simulink model "pidccontrol"  (R2014b)
settings: Solver=VariableStepAuto  StartTime=0.0  StopTime=Tstop  FixedStep=Ts  RelTol=1e-3
values from neighbouring files (symbols this model uses):
  inputnoisegain = 0    [DMCejemplo.m]
  outputnoisegain = 0    [DMCejemplo.m]
  steptimeDV = 35    [DMCejemplo.m]
  steptimeUDV = 45    [DMCejemplo.m]
  Ts = 0.5    [DMCejemplo.m]
  valueDV = 2    [DMCejemplo.m]
  valueUDV = -2    [DMCejemplo.m]
undefined symbols (not defined in the file or in its folder): Kc, Kpre, Ti
undefined symbols (not defined in the file): gdv, gu, gudv
libraries: cstblocks x3, simulink x2
settings Model: Creator=juaherdu  LastModifiedBy=juaherdu
settings DataIOCC: SaveFormat=Dataset
settings OptimizationCC: UseDivisionForNetSlopeComputation=off  SimCompilerOptimization=off
settings DebuggingCC: SolverPrmCheckMsg=none  FrameProcessingCompatibilityMsg=error  AllowSymbolicDim=off
settings HardwareCC: ProdBitPerPointer=64  ProdLargestAtomicFloat=Float  ProdIntDivRoundTo=Zero  ProdEndianess=LittleEndian  ProdWordSize=64  ProdHWDeviceType=Intel->x86-64 (Windows64)
settings RTWCC: RTWCompilerOptimization=off
settings GRTTargetCC: GeneratePreprocessorConditionals=Use local settings
settings ConfigComp: CovMetricSettings=dw  CovHtmlReporting=on  CovSaveCumulativeToWorkspaceVar=on  CovSaveSingleToWorkspaceVar=on  CovExternalEMLEnable=off

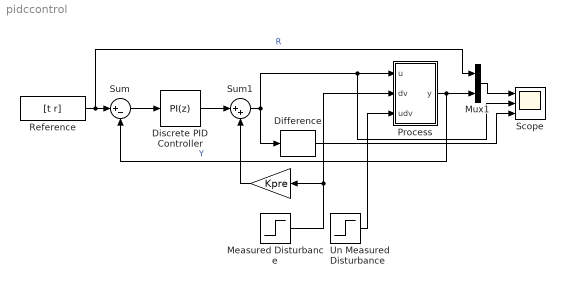
== system pidccontrol ==
  " " : Gain  Gain=Kpre
  Difference : simulink/Discrete/Difference  ICPrevInput=0.0  InputProcessing=Inherited  OutMin=[]  OutMax=[]  OutDataType=fixdt(1, 16)  OutScaling=2^-10  DoSatur=off
  Discrete PID Controller : simulink/Continuous/PID Controller  Controller=PI  TimeDomain=Discrete-time  SampleTime=Ts  IntegratorMethod=Forward Euler  FilterMethod=Forward Euler  Form=Ideal  P=Kc  I=1/Ti  D=0  N=100  InitialConditionSource=internal  InitialConditionForIntegrator=0  InitialConditionForFilter=0  ExternalReset=none  LimitOutput=off  UpperSaturationLimit=inf  LowerSaturationLimit=-inf  LinearizeAsGain=on  AntiWindupMode=none  Kb=1  TrackingMode=off  Kt=1  PParamMin=[]  PParamMax=[]  IParamMin=[]  IParamMax=[]  DParamMin=[]  DParamMax=[]  NParamMin=[]  NParamMax=[]  KbParamMin=[]  KbParamMax=[]  KtParamMin=[]  KtParamMax=[]  POutMin=[]  POutMax=[]  IOutMin=[]  IOutMax=[]  DOutMin=[]  DOutMax=[]  NOutMin=[]  NOutMax=[]  KbOutMin=[]  KbOutMax=[]  KtOutMin=[]  KtOutMax=[]  IntegratorOutMin=[]  IntegratorOutMax=[]  FilterOutMin=[]  FilterOutMax=[]  SumOutMin=[]  SumOutMax=[]  SumI1OutMin=[]  SumI1OutMax=[]  SumI2OutMin=[]  SumI2OutMax=[]  SumI3OutMin=[]  SumI3OutMax=[]  SumDOutMin=[]  SumDOutMax=[]  SaturationOutMin=[]  SaturationOutMax=[]  IntegratorContinuousStateAttributes=''  IntegratorStateMustResolveToSignalObject=off  IntegratorRTWStateStorageClass=Auto  FilterContinuousStateAttributes=''  FilterStateMustResolveToSignalObject=off  FilterRTWStateStorageClass=Auto  DifferentiatorICPrevScaledInput=0  DifferentiatorOutMin=[]  DifferentiatorOutMax=[]  UseFilter=on
  Measured Disturbance : Step  Time=steptimeDV  After=valueDV  SampleTime=Ts
  Mux1 : Mux  Inputs=2
  Process : Subsystem  mask{gu=gu, gdv=gdv, gudv=gudv, inputnoisegain=inputnoisegain, outputnoisegain=outputnoisegain}
      mask prompts: gu "fdt y/u"; gdv "fdt y/dv"; gudv "fdt y/udv"; inputnoisegain "inputnoise"; outputnoisegain "outputnoise"
      mask DialogControl DescTextVar Prompt: Parametros del Modelo del proceso
  Reference : FromWorkspace  VariableName=[t r]  SampleTime=Ts
  Scope : Scope  NumInputPorts=3
      settings: ShowLegends=on  YMin=-1.61853~-1.61915~-0.12834  YMax=14.56673~14.57238~0.68093  SaveName=Simul  MaxDataPoints=50000
  Sum : Sum  Inputs=|+-
  Sum1 : Sum  Inputs=|++
  Un Measured Disturbance : Step  Time=steptimeUDV  After=valueUDV  SampleTime=Ts
  wires:
  Measured Disturbance/1 -> " "/1, Process/2(dv)
  Un Measured Disturbance/1 -> Process/3(udv)
  Reference/1 -> Mux1/1, Sum/1  "R"
  Sum1/1 -> Scope/2, Process/1(u), Difference/1
  Process/1(y) -> Sum/2, Mux1/2  "Y"
  Mux1/1 -> Scope/1
  Difference/1 -> Scope/3
  Sum/1 -> Discrete PID Controller/1
  Discrete PID Controller/1 -> Sum1/1
  " "/1 -> Sum1/2

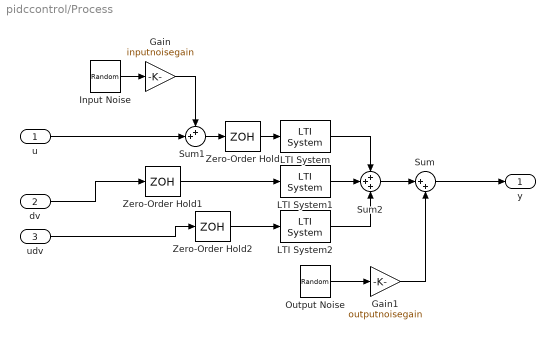
== system pidccontrol/Process ==
  u : Inport
  dv : Inport  Port=2
  udv : Inport  Port=3
  Gain : Gain  Gain=inputnoisegain
  Gain1 : Gain  Gain=outputnoisegain
  Input Noise : UniformRandomNumber  SampleTime=Ts
  LTI System : cstblocks/LTI System  sys=gu  IC=[]
  LTI System1 : cstblocks/LTI System  sys=gdv  IC=[]
  LTI System2 : cstblocks/LTI System  sys=gudv  IC=[]
  Output Noise : UniformRandomNumber  SampleTime=Ts
  Sum : Sum  Inputs=|++
  Sum1 : Sum  Inputs=++|
  Sum2 : Sum  Inputs=+++
  Zero-Order Hold : ZeroOrderHold  SampleTime=Ts
  Zero-Order Hold1 : ZeroOrderHold  SampleTime=Ts
  Zero-Order Hold2 : ZeroOrderHold  SampleTime=Ts
  y : Outport
  wires:
  Sum/1 -> y/1
  dv/1 -> Zero-Order Hold1/1
  Gain1/1 -> Sum/2
  udv/1 -> Zero-Order Hold2/1
  u/1 -> Sum1/2
  Sum2/1 -> Sum/1
  Output Noise/1 -> Gain1/1
  Input Noise/1 -> Gain/1
  Sum1/1 -> Zero-Order Hold/1
  LTI System2/1 -> Sum2/3
  LTI System/1 -> Sum2/1
  LTI System1/1 -> Sum2/2
  Gain/1 -> Sum1/1
  Zero-Order Hold/1 -> LTI System/1
  Zero-Order Hold1/1 -> LTI System1/1
  Zero-Order Hold2/1 -> LTI System2/1
